simulink model "DynamicModel"  (R2022a)
settings: Solver=ode4  StartTime=0.0  StopTime=20  FixedStep=1e-3  MaxStep=1e-5  RelTol=1e-3
InitFcn:
  | SM_Data_static
StopFcn:
  | filename='forPlot'
  | forPlot
values from neighbouring files (symbols this model uses):
  d_Phi_b = [0,0,0].'    [SM_Data_static.m]
  d_theta_m = [0,0,0,0].'    [SM_Data_static.m]
  H_b = [1.2,0,-0.3;1,0.89,0.24;0.36,0,0.21]    [SM_Data_static.m]
  Kdbf = diag([1.2,2.1,1.5],0)    [SM_Data_static.m]
  Kdmf = diag([0.65,0.89,0.99,1.2],0)    [SM_Data_static.m]
  Kibc = diag([1.1,1.3,1.5],0)    [SM_Data_static.m]
  Kimc = diag([0.88,0.86,0.75,0.89],0)    [SM_Data_static.m]
  Kpbc = -diag([5,5,4.8],0)    [SM_Data_static.m]
  Kpbf = diag([3.2,3.4,5.2],0)    [SM_Data_static.m]
  Kpmc = -diag([5.2,4.3,6.5,4.8],0)    [SM_Data_static.m]
  Kpmf = diag([4,3,6,5],0)    [SM_Data_static.m]
  M_m = [3.125,0,0,0 ... (first row only)    [SM_Data_static.m]
  M_mw = M_wm'    [SM_Data_static.m]
  M_w = [6891,0,0 ... (first row only)    [SM_Data_static.m]
  M_wm = [10,0,0,0 ... (first row only)    [SM_Data_static.m]
  Phi_b = [0.8,-0.6,0.5].'    [SM_Data_static.m]
  Phi_b_d = [0.2,0.1,0.3].'    [SM_Data_static.m]
  theta_m = [1.5,0.7,1.0,2.3].'    [SM_Data_static.m]
  theta_m_d = [0.3,0.4,0.5,0.6].'    [SM_Data_static.m]
settings Model: Creator=Zou Xiangxiang  LastModifiedBy=43840

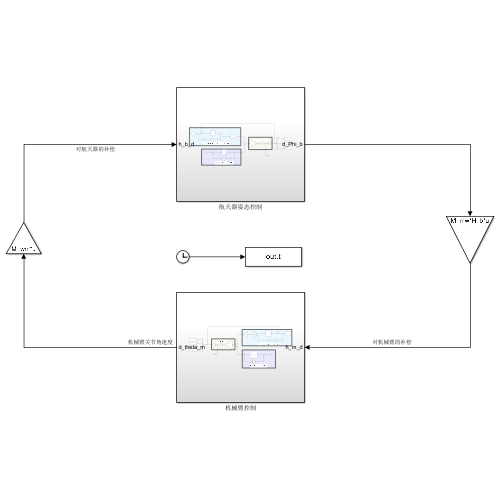
[thumbnail: Simulink's stored preview of the top-level diagram]
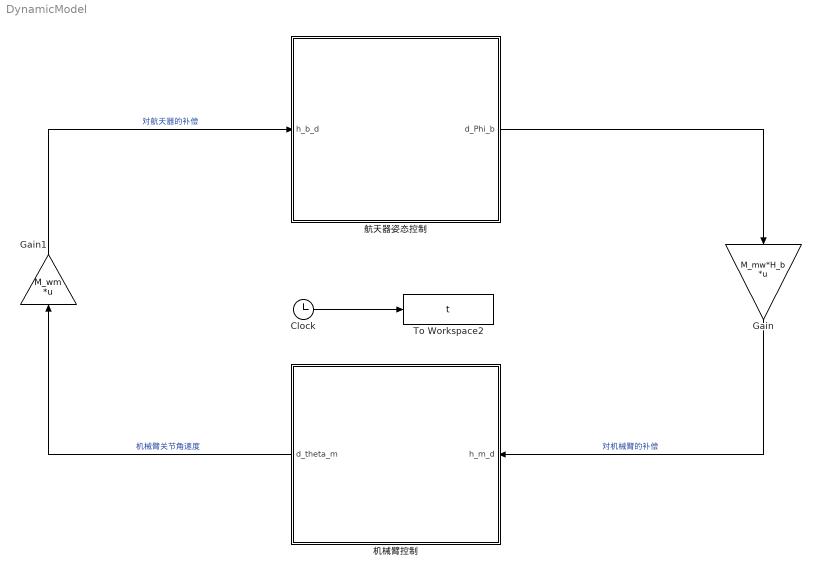
== system DynamicModel ==
  Clock : Clock
  Gain : Gain  Gain=M_mw*H_b  Multiplication=Matrix(K*u)
  Gain1 : Gain  Gain=M_wm  Multiplication=Matrix(K*u)
  To Workspace2 : ToWorkspace  VariableName=t  SampleTime=-1
      settings: Save2DSignal=2-D array (concatenate along first dimension)
  机械臂控制 : Subsystem
  航天器姿态控制 : Subsystem
  wires:
  Gain1/1 -> 航天器姿态控制/1(h_b_d)  "对航天器的补偿"
  Gain/1 -> 机械臂控制/1(h_m_d)  "对机械臂的补偿"
  机械臂控制/1(d_theta_m) -> Gain1/1  "机械臂关节角速度"
  Clock/1 -> To Workspace2/1
  航天器姿态控制/1(d_Phi_b) -> Gain/1

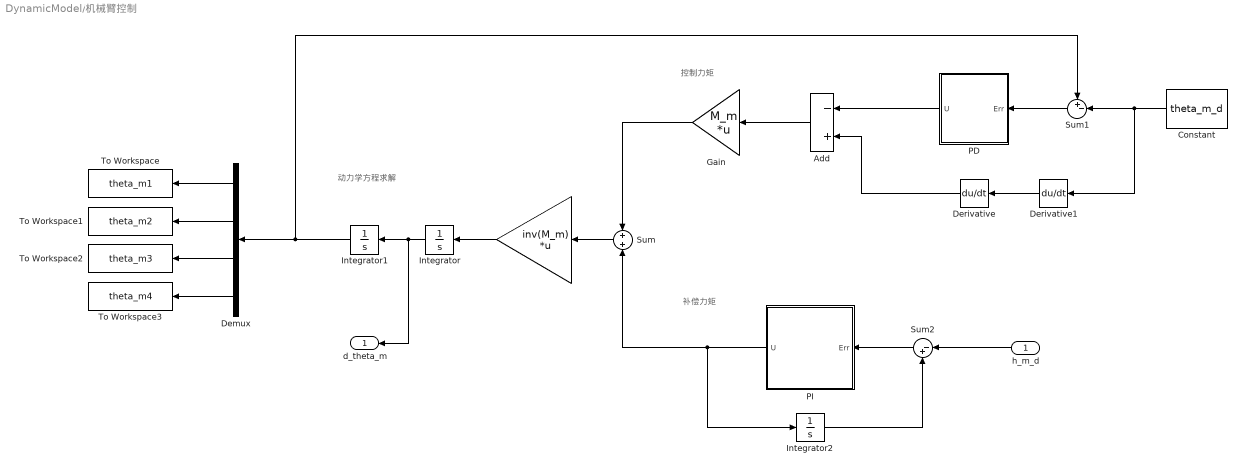
== system DynamicModel/机械臂控制 ==
  note: 动力学方程求解
  note: 控制力矩
  note: 补偿力矩
  h_m_d : Inport
  " " : Gain  Gain=inv(M_m)  Multiplication=Matrix(K*u)
  Add : Sum  Inputs=-+
  Constant : Constant  Value=theta_m_d
  Demux : Demux
  Derivative : Derivative
  Derivative1 : Derivative
  Gain : Gain  Gain=M_m  Multiplication=Matrix(K*u)
  Integrator : Integrator  InitialCondition=d_theta_m
  Integrator1 : Integrator  InitialCondition=theta_m
  Integrator2 : Integrator
  PD : Subsystem
  PI : Subsystem
  Sum : Sum  Inputs=+|+
  Sum1 : Sum  Inputs=+-|
  Sum2 : Sum  Inputs=|-+
  To Workspace : ToWorkspace  VariableName=theta_m1  SampleTime=-1
      settings: Save2DSignal=2-D array (concatenate along first dimension)
  To Workspace1 : ToWorkspace  VariableName=theta_m2  SampleTime=-1
      settings: Save2DSignal=2-D array (concatenate along first dimension)
  To Workspace2 : ToWorkspace  VariableName=theta_m3  SampleTime=-1
      settings: Save2DSignal=2-D array (concatenate along first dimension)
  To Workspace3 : ToWorkspace  VariableName=theta_m4  SampleTime=-1
      settings: Save2DSignal=2-D array (concatenate along first dimension)
  d_theta_m : Outport
  wires:
  Integrator2/1 -> Sum2/2
  Integrator/1 -> Integrator1/1, d_theta_m/1
  PI/1(U) -> Sum/2, Integrator2/1
  Sum/1 -> " "/1
  Sum2/1 -> PI/1(Err)
  " "/1 -> Integrator/1
  Constant/1 -> Sum1/2, Derivative1/1
  Derivative1/1 -> Derivative/1
  Sum1/1 -> PD/1(Err)
  Gain/1 -> Sum/1
  Add/1 -> Gain/1
  PD/1(U) -> Add/1
  Derivative/1 -> Add/2
  h_m_d/1 -> Sum2/1
  Integrator1/1 -> Demux/1, Sum1/1
  Demux/1 -> To Workspace/1
  Demux/2 -> To Workspace1/1
  Demux/3 -> To Workspace2/1
  Demux/4 -> To Workspace3/1

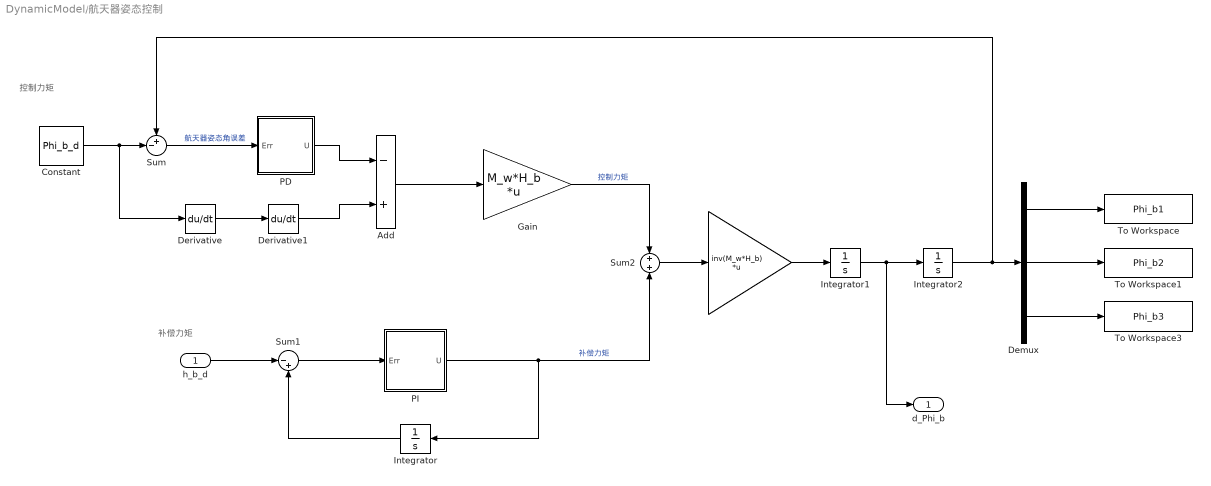
== system DynamicModel/航天器姿态控制 ==
  note: 补偿力矩
  note: 控制力矩
  h_b_d : Inport
  " " : Gain  Gain=inv(M_w*H_b)  Multiplication=Matrix(K*u)
  Add : Sum  Inputs=-+
  Constant : Constant  Value=Phi_b_d  VectorParams1D=off
  Demux : Demux  Outputs=3
  Derivative : Derivative
  Derivative1 : Derivative
  Gain : Gain  Gain=M_w*H_b  Multiplication=Matrix(K*u)
  Integrator : Integrator
  Integrator1 : Integrator  InitialCondition=d_Phi_b
  Integrator2 : Integrator  InitialCondition=Phi_b
  PD : Subsystem
  PI : Subsystem
  Sum : Sum  Inputs=+-|
  Sum1 : Sum  Inputs=|-+
  Sum2 : Sum  Inputs=+|+
  To Workspace : ToWorkspace  VariableName=Phi_b1  SampleTime=-1
      settings: Save2DSignal=2-D array (concatenate along first dimension)
  To Workspace1 : ToWorkspace  VariableName=Phi_b2  SampleTime=-1
      settings: Save2DSignal=2-D array (concatenate along first dimension)
  To Workspace3 : ToWorkspace  VariableName=Phi_b3  SampleTime=-1
      settings: Save2DSignal=2-D array (concatenate along first dimension)
  d_Phi_b : Outport
  wires:
  Sum/1 -> PD/1(Err)  "航天器姿态角误差"
  Integrator/1 -> Sum1/2
  " "/1 -> Integrator1/1
  Sum1/1 -> PI/1(Err)
  Derivative/1 -> Derivative1/1
  Gain/1 -> Sum2/1  "控制力矩"
  PD/1(U) -> Add/1
  Add/1 -> Gain/1
  Sum2/1 -> " "/1
  PI/1(U) -> Sum2/2, Integrator/1  "补偿力矩"
  h_b_d/1 -> Sum1/1
  Integrator1/1 -> d_Phi_b/1, Integrator2/1
  Derivative1/1 -> Add/2
  Constant/1 -> Derivative/1, Sum/2
  Integrator2/1 -> Sum/1, Demux/1
  Demux/1 -> To Workspace/1
  Demux/2 -> To Workspace1/1
  Demux/3 -> To Workspace3/1

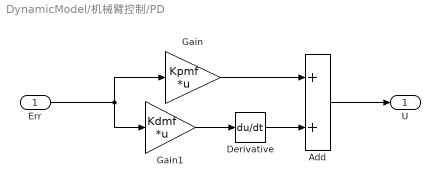
== system DynamicModel/机械臂控制/PD ==
  Err : Inport
  Add : Sum
  Derivative : Derivative
  Gain : Gain  Gain=Kpmf  Multiplication=Matrix(K*u)
  Gain1 : Gain  Gain=Kdmf  Multiplication=Matrix(K*u)
  U : Outport
  wires:
  Err/1 -> Gain1/1, Gain/1
  Gain1/1 -> Derivative/1
  Gain/1 -> Add/1
  Derivative/1 -> Add/2
  Add/1 -> U/1

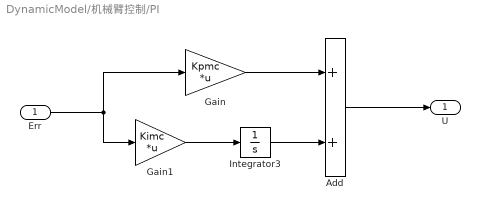
== system DynamicModel/机械臂控制/PI ==
  Err : Inport
  Add : Sum
  Gain : Gain  Gain=Kpmc  Multiplication=Matrix(K*u)
  Gain1 : Gain  Gain=Kimc  Multiplication=Matrix(K*u)
  Integrator3 : Integrator
  U : Outport
  wires:
  Gain1/1 -> Integrator3/1
  Add/1 -> U/1
  Gain/1 -> Add/1
  Err/1 -> Gain1/1, Gain/1
  Integrator3/1 -> Add/2

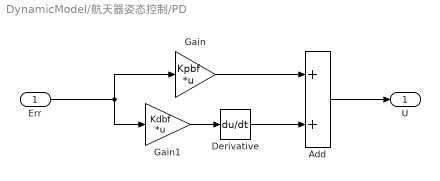
== system DynamicModel/航天器姿态控制/PD ==
  Err : Inport
  Add : Sum
  Derivative : Derivative
  Gain : Gain  Gain=Kpbf  Multiplication=Matrix(K*u)
  Gain1 : Gain  Gain=Kdbf  Multiplication=Matrix(K*u)
  U : Outport
  wires:
  Err/1 -> Gain1/1, Gain/1
  Gain1/1 -> Derivative/1
  Gain/1 -> Add/1
  Derivative/1 -> Add/2
  Add/1 -> U/1

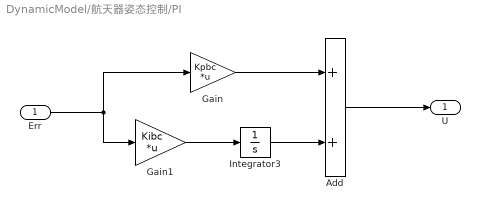
== system DynamicModel/航天器姿态控制/PI ==
  Err : Inport
  Add : Sum
  Gain : Gain  Gain=Kpbc  Multiplication=Matrix(K*u)
  Gain1 : Gain  Gain=Kibc  Multiplication=Matrix(K*u)
  Integrator3 : Integrator
  U : Outport
  wires:
  Gain1/1 -> Integrator3/1
  Add/1 -> U/1
  Gain/1 -> Add/1
  Err/1 -> Gain1/1, Gain/1
  Integrator3/1 -> Add/2
